simulink model "V2"  (Simulink 8.9)
settings: Solver=VariableStepAuto  StartTime=0.0  StopTime=20  RelTol=1e-3
values from neighbouring files (symbols this model uses):
  Fz = m*g/2    (= 3924)    [variabeln.m]    (also in variabeln_v2.m)
  J = 1    [variabeln.m]    (also in variabeln_v2.m)
  kp = 1000    [variabeln_v2.m]
  m = 800    [variabeln.m]    (also in variabeln_v2.m)
  r = 0.25    [variabeln.m]    (also in variabeln_v2.m)
  Td = 0    [variabeln_v2.m]
  theta1 = 1.28    [variabeln.m]    (also in variabeln_v2.m)
  theta2 = 23.99    [variabeln.m]    (also in variabeln_v2.m)
  theta3 = 0.52    [variabeln.m]    (also in variabeln_v2.m)
  Ti = 1    [variabeln_v2.m]
  v0 = 10    [variabeln.m]    (also in variabeln_v2.m = 50)
settings Model: LogicAnalyzerSignalOrdering=7a84ea7f-8162-432b-9086-2b07596e42c8,87e14077-1fe2-4718-b6ab-8f0f0900bfb6,b904f77b-e792-4738-9803-7afcceeeab1e,e2db8135-5d07-4714-816b-861e936b510f  Creator=frede  LastModifiedBy=Dominic
settings DataIOCC: LimitDataPoints=off  SaveFormat=Dataset  SignalLoggingSaveFormat=Dataset
settings OptimizationCC: LifeSpan=auto
settings DebuggingCC: UnderspecifiedInitializationDetection=Simplified  MergeDetectMultiDrivingBlocksExec=error  FcnCallInpInsideContextMsg=error  StateNameClashWarn=none  SFUnexpectedBacktrackingDiag=error  SFNoUnconditionalDefaultTransitionDiag=error  SFExecutionAtInitializationDiag=warning
settings HardwareCC: ProdBitPerPointer=64  ProdBitPerSizeT=64  ProdBitPerPtrDiffT=64  ProdLargestAtomicFloat=Float  ProdIntDivRoundTo=Zero  ProdEndianess=LittleEndian  ProdWordSize=64  ProdHWDeviceType=Intel->x86-64 (Windows64)
settings ModelReferenceCC: PropagateSignalLabelsOutOfModel=on
settings GRTTargetCC: TargetLangStandard=C99 (ISO)  GeneratePreprocessorConditionals=Use local settings  CombineOutputUpdateFcns=on  GRTInterface=off
settings ConfigComp: CovMetricSettings=dwe  CovHtmlReporting=off  CovSaveCumulativeToWorkspaceVar=off  CovSaveSingleToWorkspaceVar=off  CovExternalEMLEnable=on

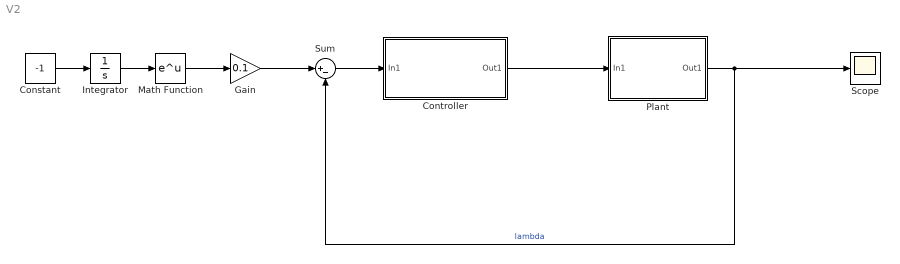
== system V2 ==
  Constant : Constant  Value=-1
  "Controller " : Subsystem
  Gain : Gain  Gain=0.1
  Integrator : Integrator
  Math Function : Math  SaturateOnIntegerOverflow=on
  Plant : Subsystem
  Scope : Scope
  Sum : Sum  Inputs=|+-
  wires:
  Math Function/1 -> Gain/1
  Plant/1(Out1) -> Scope/1, Sum/2  "lambda"
  Sum/1 -> "Controller "/1(In1)
  "Controller "/1(Out1) -> Plant/1(In1)
  Integrator/1 -> Math Function/1
  Constant/1 -> Integrator/1
  Gain/1 -> Sum/1

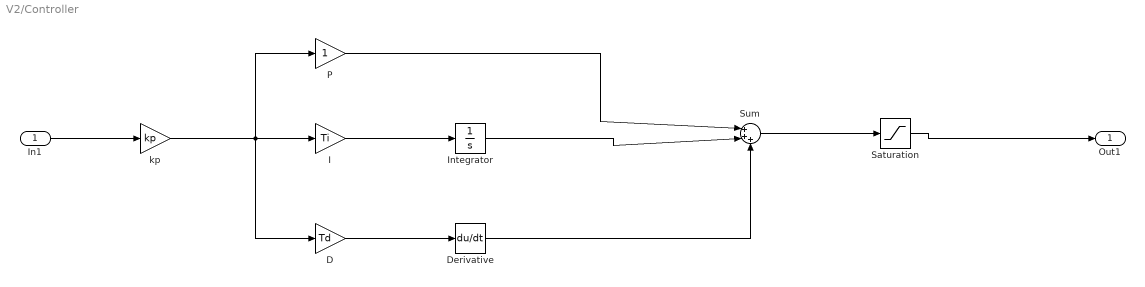
== system V2/Controller  ==
  In1 : Inport
  D : Gain  Gain=Td
  Derivative : Derivative
  I : Gain  Gain=Ti
  Integrator : Integrator
  P : Gain
  Saturation : Saturate  UpperLimit=140  LowerLimit=0
  Sum : Sum  Inputs=|+++
  kp : Gain  Gain=kp
  Out1 : Outport
  wires:
  D/1 -> Derivative/1
  I/1 -> Integrator/1
  P/1 -> Sum/1
  Integrator/1 -> Sum/2
  Derivative/1 -> Sum/3
  kp/1 -> D/1, P/1, I/1
  In1/1 -> kp/1
  Sum/1 -> Saturation/1
  Saturation/1 -> Out1/1

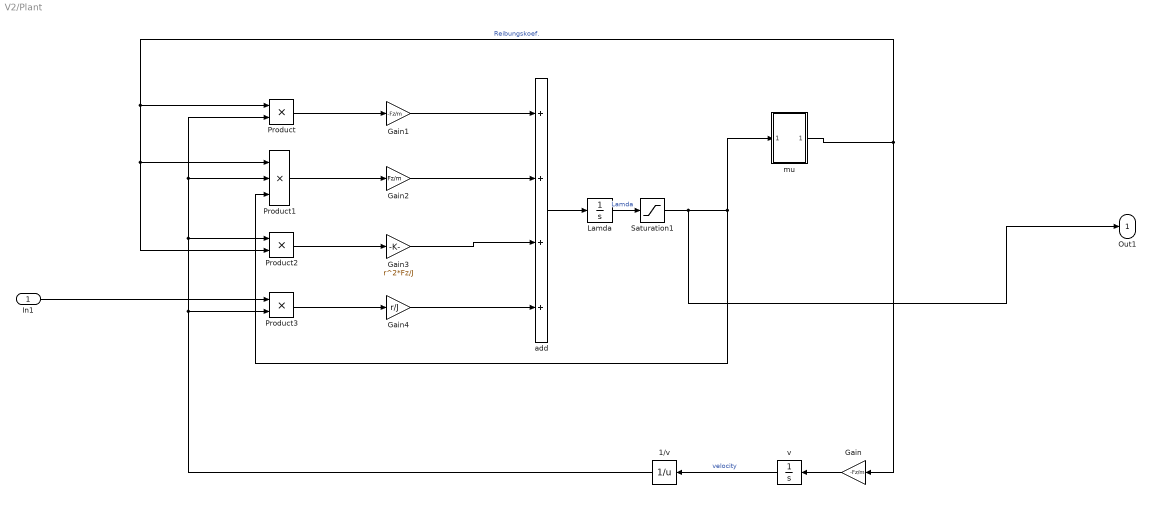
== system V2/Plant ==
  In1 : Inport
  "1/v " : Math  Operator=reciprocal  SaturateOnIntegerOverflow=on
  Gain : Gain  Gain=-Fz/m
  Gain1 : Gain  Gain=-Fz/m
  Gain2 : Gain  Gain=Fz/m
  Gain3 : Gain  Gain=r^2*Fz/J
  Gain4 : Gain  Gain=r/J
  Lamda : Integrator  IgnoreLimit=on
  Product : Product
  Product1 : Product  Inputs=3
  Product2 : Product
  Product3 : Product
  Saturation1 : Saturate  UpperLimit=1  LowerLimit=0
  add : Sum  Inputs=++++
  mu : Subsystem
  v : Integrator  InitialCondition=v0
  Out1 : Outport
  wires:
  v/1 -> "1/v "/1  "velocity"
  Product2/1 -> Gain3/1
  "1/v "/1 -> Product3/2, Product2/1, Product1/2, Product/2
  Gain/1 -> v/1
  Product3/1 -> Gain4/1
  Gain4/1 -> add/4
  Product/1 -> Gain1/1
  Gain3/1 -> add/3
  Gain2/1 -> add/2
  Product1/1 -> Gain2/1
  Gain1/1 -> add/1
  add/1 -> Lamda/1
  mu/1(Out1) -> Product2/2, Product1/1, Product/1, Gain/1  "Reibungskoef."
  In1/1 -> Product3/1
  Lamda/1 -> Saturation1/1  "Lamda"
  Saturation1/1 -> Out1/1, Product1/3, mu/1(In1)

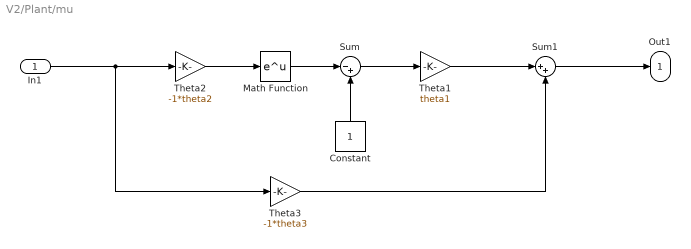
== system V2/Plant/mu ==
  In1 : Inport
  Constant : Constant
  Math Function : Math  SaturateOnIntegerOverflow=on
  Sum : Sum  Inputs=|-+
  Sum1 : Sum  Inputs=|++
  Theta1 : Gain  Gain=theta1
  "Theta2 " : Gain  Gain=-1*theta2
  "Theta3 " : Gain  Gain=-1*theta3
  Out1 : Outport
  wires:
  In1/1 -> "Theta3 "/1, "Theta2 "/1
  Math Function/1 -> Sum/1
  Sum/1 -> Theta1/1
  "Theta3 "/1 -> Sum1/2
  Theta1/1 -> Sum1/1
  Sum1/1 -> Out1/1
  "Theta2 "/1 -> Math Function/1
  Constant/1 -> Sum/2
